simulink model "IQ_GEN"  (R2024a)
settings: Solver=VariableStepAuto  StartTime=0.0  StopTime=10.0  RelTol=1e-3
settings Model: Creator=cian.odonnell  LastModifiedBy=cian.odonnell

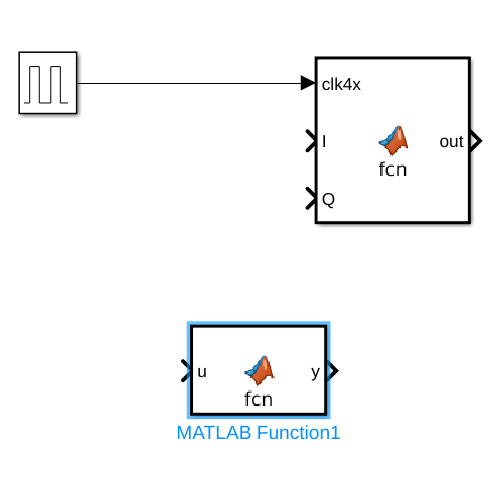
[thumbnail: Simulink's stored preview of the top-level diagram]
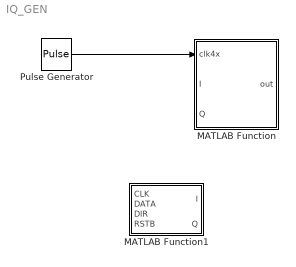
== system IQ_GEN ==
  MATLAB Function : MATLAB Function  TreatAsAtomicUnit=on
  MATLAB Function1 : MATLAB Function  TreatAsAtomicUnit=on
  Pulse Generator : DiscretePulseGenerator  PulseType=Time based  Period=1/(4e6)  PulseWidth=50
  wires:
  Pulse Generator/1 -> MATLAB Function/1(clk4x)

== matlab function IQ_GEN/MATLAB Function1 ==
  data: CLK input; I output; DATA input; DIR input; RSTB input; Q output
function [I, Q] = DATA_MODULATOR(CLK, DATA, DIR, RSTB)
    % Internal State Mapping: 
    % 0: 0°, 1: 90°, 2: 180°, 3: 270°
    persistent state;
    if isempty(state)
        state = uint8(0); 
    end

    persistent last_clk;
    if isempty(last_clk)
        last_clk = false;
    end

    % 1. Synchronous Control Logic (1MHz Domain)
    if (CLK && ~last_clk)
        
        % RSTB (Active-Low): 0 = Reset, 1 = Normal Operation
        if RSTB == 0
            state = uint8(0); % Force constellation to 0°
        elseif DATA == 1
            % Trigger phase shift on DATA pulse
            if DIR == 1
                % Lead (+90°)
                state = mod(state + 1, 4);
            else
                % Lag (-90°)
                if state == 0
                    state = uint8(3);
                else
                    state = state - 1;
                end
            end
        end
        
    end
    last_clk = CLK;

    % 2. Constellation Mapping (Gray Code Selection)
    % These bits act as the address for your 4:1 Phase MUX
    switch state
        case 0 % 0°
            I = false; Q = false;
        case 1 % 90°
            I = false; Q = true;
        case 2 % 180°
            I = true;  Q = true;
        case 3 % 270°
            I = true;  Q = false;
    end
end

== matlab function IQ_GEN/MATLAB Function ==
  data: clk4x input; I input; out output; Q input
function out = fcn(clk4x, I, Q)
    % persistent variables to track state and detect edges
    persistent count;
    if isempty(count)
        count = uint8(0);
    end
    
    persistent last_clk;
    if isempty(last_clk)
        last_clk = false;
    end

    % 1. Synchronous Counter (Divide by 4)
    % Increments on the rising edge of the 4x clock
    if (clk4x && ~last_clk)
        count = mod(count + 1, 4);
    end
    last_clk = clk4x;

    % 2. Generate the 4 Quadrature Phases (1 MHz)
    % These are derived from the 4-state counter
    % ph0:  1 1 0 0 (State 0,1)
    % ph90: 0 1 1 0 (State 1,2)
    ph0   = (count == 0 || count == 1); 
    ph90  = (count == 1 || count == 2);
    ph180 = ~ph0;
    ph270 = ~ph90;

    % 3. 4:1 Multiplexer Logic
    % Uses I and Q as the selection bits
    if (~I && ~Q)
        out = ph0;   % 00 -> 0°
    elseif (~I && Q)
        out = ph90;  % 01 -> 90°
    elseif (I && ~Q)
        out = ph180; % 10 -> 180°
    else
        out = ph270; % 11 -> 270°
    end
end
